simulink model "aufgabe_3_1"  (R2017b)
settings: Solver=ode5  StartTime=0.0  StopTime=0.3  FixedStep=10e-6  RelTol=1e-3
values from neighbouring files (symbols this model uses):
  Cr = ((km*i)-Mm(:,4))./W(:,4)    [aufgabe2_cr.m]    (also in aufgabe3.m = 5e-06; aufgabe4.m = 5e-06; aufgabe6.m = 5e-06)
  J = 0.5e-6    (= 5e-07)    [aufgabe3.m]    (also in aufgabe4.m = 3e-06; aufgabe6.m = 3e-06)
  ke = 0.024    [aufgabe2_cr.m]    (also in aufgabe3.m; aufgabe4.m; aufgabe6.m)
  km = 0.0232    [aufgabe2_cr.m]    (also in aufgabe3.m = 0.0227; aufgabe4.m = 0.023; aufgabe6.m = 0.023)
  L = Lm+Ls    [aufgabe2.m]    (also in aufgabe2_cr.m = 0.0004; aufgabe3.m = 0.0004; aufgabe4.m = 0.0004; aufgabe6.m = 0.0004)
  Ml = 0    [aufgabe2_cr.m]    (also in aufgabe3.m; aufgabe6.m)
  R = 3+(2*rand-1)*0.4    [aufgabe1.m]    (also in aufgabe2.m = 3; aufgabe2_cr.m = 3; aufgabe3.m = 3; aufgabe4.m = 3)
  U0 = 12    [aufgabe2_cr.m]    (also in aufgabe3.m; aufgabe4.m = 20; aufgabe6.m)
settings Model: Creator=gurbuz  LastModifiedBy=gurbuz

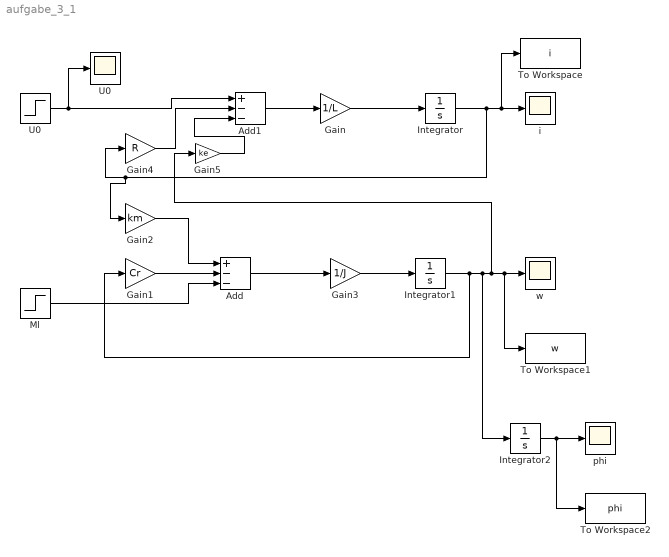
== system aufgabe_3_1 ==
  Add : Sum  Inputs=+--
  Add1 : Sum  Inputs=+--
  Gain : Gain  Gain=1/L
  Gain1 : Gain  Gain=Cr
  Gain2 : Gain  Gain=km
  Gain3 : Gain  Gain=1/J
  Gain4 : Gain  Gain=R
  Gain5 : Gain  Gain=ke
  Integrator : Integrator
  Integrator1 : Integrator
  Integrator2 : Integrator
  "Ml " : Step  Time=0  After=Ml  SampleTime=0
  To Workspace : ToWorkspace  VariableName=i  SaveFormat=Timeseries  SampleTime=-1
  To Workspace1 : ToWorkspace  VariableName=w  SaveFormat=Timeseries  SampleTime=-1
  To Workspace2 : ToWorkspace  VariableName=phi  SaveFormat=Timeseries  SampleTime=-1
  "U0 " : Step  Time=0.1  After=U0  SampleTime=0
  "U0 " : Scope
  "i " : Scope
  "phi " : Scope
  "w " : Scope
  wires:
  "U0 "/1 -> Add1/1, "U0 "/1
  Add1/1 -> Gain/1
  Gain/1 -> Integrator/1
  Integrator/1 -> Gain2/1, Gain4/1, To Workspace/1, "i "/1
  Add/1 -> Gain3/1
  Gain3/1 -> Integrator1/1
  Integrator1/1 -> Gain1/1, Integrator2/1, Gain5/1, To Workspace1/1, "w "/1
  Gain2/1 -> Add/1
  Gain1/1 -> Add/2
  "Ml "/1 -> Add/3
  Gain5/1 -> Add1/3
  Gain4/1 -> Add1/2
  Integrator2/1 -> To Workspace2/1, "phi "/1
